simulink model "dynamicANN"  (R2019b)
settings: Solver=VariableStepAuto  StartTime=0.0  StopTime=3  RelTol=1e-3
values from neighbouring files (symbols this model uses):
  a = 87.548e-3    (= 0.087548)    [main.m]
  b = 132.452e-3    (= 0.132452)    [main.m]
  d = 22.452e-3    (= 0.022452)    [main.m]
  delta = 4e-6    (= 4e-06)    [main.m]
  F1 = mass*g-F2    (= 23.4474357109)    [main.m]
  F2 = a*mass*g/(a+b)    (= 15.4982642891)    [main.m]
  g = 9.81    [main.m]
  h0 = 75e-6    (= 7.5e-05)    [main.m]
  Jd = 0.047331604    [main.m]
  Jp = 0.00075    [main.m]
  Kps = (Vmax-Vmin)/(Hmax-Hmin)    (= 1666.66666667)    [main.m]
  Ksv = 30    [main.m]
  mass = 3.970    (= 3.97)    [main.m]
  mm = F2/g    (= 1.57984345455)    [main.m]
  omega = n_rpm*2*pi/60    (= 293.215314335)    [main.m]
  s = 30e-3    (= 0.03)    [main.m]
  tau = 0.12    [main.m]
  taus = 0.00125    [main.m]
  Ts = 1/fs    (= 0.001)    [main.m]
libraries: neural x480, simulink x2
(part 11 of 11)

== system dynamicANN/SERVOVALVES/HYDROSTATIC FORCES APPROXIMATION/Layer 2/LW{2,1} ==
  "ad{2,1}" : Inport  PortDimensions=50
      mask Display: e = 0.06;c1 = [120 230 180]/255;c2 = ([120 230 180]+0)/(256+128);c3 = ([120 230 180]+128)/(256+128);patch([0 1 1 0],[0 0 1 1],c1);patch([0 1 1 1-e 1-e 0+e],[0 0 1 1-e 0+e 0+e],c2);patch([0 0 1 1-e 0+e 0+e],[0 1 1 1-e 1-e 0+e],c3);plot([0 1 1 0 0],[0 0 1 1 0]);
  "IW{2,1}(1,:)'" : Constant  Value=[-1.014165171456560710083749654586426913738250732421875;0.74254120405114820702152655940153636038303375244140625;-0.493657103560888099735848300042562186717987060546875;1.762347654234217575464072069735266268253326416015625;0.77261513991503283360628984155482612550258636474609375;0.318276655083587822758772745146416127681732177734375;0.4305854427140574092192082389374263584613800048828125;0.1184731097225189266897160678126965649425983428955078125;-0.438124466002386803165080664257402531802654266357421875;1.09137751006303229672766974545083940029144287109375;-0.490669166841488202379650829243473708629608154296875;-0.98834811164750779877152808694518171250820159912109375;1.0590431490617298049272676507825963199138641357421875;-1.776082676108671432047003690968267619609832763671875;-2.06612743120169906063665621331892907619476318359375;-0.64589634160559905584619855289929546415805816650390625;-0.4327766588303278982863275814452208578586578369140625;-1.727153899806108672265736458939500153064727783203125;0.59181904704496124391965850009000860154628753662109375;0.16959741359399671534191611499409191310405731201171875;0.67424149151247203537451468946528621017932891845703125;0.585530221611660461888959616771899163722991943359375;1.0280769199996886431591747168567962944507598876953125;-0.2953895750385611140842456734389998018741607666015625;-0.288245131766746875978668640527757816016674041748046875;1.3110256721162059090346474476973526179790496826171875;-0.94479089477446398515070313806063495576381683349609375;2.976859202869103881994305993430316448211669921875;1.00813878716374727417814938235096633434295654296875;0.55045191126284465088502884100307710468769073486328125;-0.402896139933797303722684546301024965941905975341796875;0.6531782510692634158289138213149271905422210693359375;-0.339620575450382045090691462974064052104949951171875;-1.548768075257708431990977260284125804901123046875;-0.1751011740113746217861745435584452934563159942626953125;-1.493850957399413648118979835999198257923126220703125;-0.414405881298872402762611955040483735501766204833984375;1.3784631005445773244133533808053471148014068603515625;0.43496611827169628927691746866912581026554107666015625;1.2371551637692241865096320907468907535076141357421875;-0.429415029853276120075378230467322282493114471435546875;0.72610511484034712115231968709849752485752105712890625;0.528784547083847922266386376577429473400115966796875;-0.355625475679885505453370342365815304219722747802734375;-0.81546763135191124849399102458846755325794219970703125;-0.43196629902076733031890398706309497356414794921875;2.141633472647410219025232436251826584339141845703125;-0.942809116362634203056813930743373930454254150390625;0.50673484573840033018399253705865703523159027099609375;-0.311824293494437132512331345424172468483448028564453125]
      mask Display: e = 0.06;c1 = [120 150 230]/255;c2 = ([120 150 230]+0)/383;c3 = ([120 150 230]+128)/383;patch([0 1 1 0],[0 0 1 1],c1);patch([0 1 1 1-e 1-e 0+e],[0 0 1 1-e 0+e 0+e],c2);patch([0 0 1 1-e 0+e 0+e],[0 1 1 1-e 1-e 0+e],c3);plot([0 1 1 0 0],[0 0 1 1 0]);disp('weights');
  "IW{2,1}(2,:)'" : Constant  Value=[3.02639673612086568255108431912958621978759765625;0.7885923810484214424576521196286194026470184326171875;-2.164530907189261110801226095645688474178314208984375;-0.245729748797801850201949491747654974460601806640625;-0.00808531557296920423694164270500550628639757633209228515625;-0.76387022351862265967525900123291648924350738525390625;0.0827290827070368550710810495729674585163593292236328125;-0.6097012388277927019686330822878517210483551025390625;-0.74928046916180968128884387624566443264484405517578125;2.951882377774577737028494084370322525501251220703125;-2.1842359326909264183314007823355495929718017578125;2.530648543456691879072195661137811839580535888671875;3.18021236840055276928751482046209275722503662109375;0.14051115708063510734149303971207700669765472412109375;0.06445474728021070853767326980232610367238521575927734375;1.457545283477658326631853924482129514217376708984375;-1.621429868292408205121546416194178164005279541015625;0.279376315092421834140878900143434293568134307861328125;-0.8789785739954181220667805973789654672145843505859375;1.3220455668841974983251930098049342632293701171875;1.933304350227246004578773863613605499267578125;1.098485890073359172447453602217137813568115234375;-1.50724817303466007700762929744087159633636474609375;-0.6862057691770095946282026488916017115116119384765625;-1.1824579770952807766803971389890648424625396728515625;-1.294521403451049490485047499532811343669891357421875;0.435494894476214755574261516812839545309543609619140625;-1.1980880870527113035706179289263673126697540283203125;-0.29411642131463688887293983498238958418369293212890625;-0.5801295069320904218557188869453966617584228515625;0.00783844178986191353342150023308931849896907806396484375;0.64151166497871681126952125850948505103588104248046875;-0.580909108960366182827783632092177867889404296875;-1.5317767480030484161801496156840585172176361083984375;-1.55665554144854834106581620289944112300872802734375;-1.444847369615960275268662371672689914703369140625;-1.3425084490430860828524828320951201021671295166015625;-0.5131835470496282081143135656020604074001312255859375;0.764211347515264538543533490155823528766632080078125;-0.1667272900532859314370881520517286844551563262939453125;1.6458130141065983043091591753182001411914825439453125;-0.2219392160808244252034882038060459308326244354248046875;1.6264036561568058214533039063098840415477752685546875;-0.18886871647990266520622526513761840760707855224609375;-0.728706117737796699174168679746799170970916748046875;-2.016403595037946860912825286504812538623809814453125;0.029398033365513019654624571330714388750493526458740234375;-2.93245822543744250054942312999628484249114990234375;3.147405101749385369913625254412181675434112548828125;1.4208462681749429723510047551826573908329010009765625]
      mask Display: e = 0.06;c1 = [120 150 230]/255;c2 = ([120 150 230]+0)/383;c3 = ([120 150 230]+128)/383;patch([0 1 1 0],[0 0 1 1],c1);patch([0 1 1 1-e 1-e 0+e],[0 0 1 1-e 0+e 0+e],c2);patch([0 0 1 1-e 0+e 0+e],[0 1 1 1-e 1-e 0+e],c3);plot([0 1 1 0 0],[0 0 1 1 0]);disp('weights');
  Mux : Mux  Inputs=2
      mask Display: e = 0.06;c1 = [120 150 230]/255;c2 = ([120 150 230]+0)/383;c3 = ([120 150 230]+128)/383;patch([0 1 1 0],[0 0 1 1],c1);patch([0 1 1 1-e 1-e 0+e],[0 0 1 1-e 0+e 0+e],c2);patch([0 0 1 1-e 0+e 0+e],[0 1 1 1-e 1-e 0+e],c3);plot([0 1 1 0 0],[0 0 1 1 0]);disp('Mux');
  dotprod1 : neural/Weight Functions/dotprod
      settings: SourceProductName=Deep Learning Toolbox
  dotprod2 : neural/Weight Functions/dotprod
      settings: SourceProductName=Deep Learning Toolbox
  "lz{2,1}" : Outport
      mask Display: e = 0.06;c1 = [120 230 180]/255;c2 = ([120 230 180]+0)/(256+128);c3 = ([120 230 180]+128)/(256+128);patch([0 1 1 0],[0 0 1 1],c1);patch([0 1 1 1-e 1-e 0+e],[0 0 1 1-e 0+e 0+e],c2);patch([0 0 1 1-e 0+e 0+e],[0 1 1 1-e 1-e 0+e],c3);plot([0 1 1 0 0],[0 0 1 1 0]);
  wires:
  "IW{2,1}(1,:)'"/1 -> dotprod1/1
  "ad{2,1}"/1 -> dotprod1/2, dotprod2/2
  dotprod1/1 -> Mux/1
  "IW{2,1}(2,:)'"/1 -> dotprod2/1
  dotprod2/1 -> Mux/2
  Mux/1 -> "lz{2,1}"/1

== matlab function dynamicANN/REFERENCE SHAPING (cos) ==
  data: t input; t0 input; t1 input; Xc input; REFX output; Yc input; Xref input; Yref input; REFY output
function [REFX, REFY] = RefShaping(t,t0,t1,Xc,Yc,Xref,Yref)
Ax=(Xref-Xc)/2;
Ay=(Yref-Yc)/2;
w=pi/(t1-t0);

if t<t0
    REFX=Xc;
    REFY=Yc;
else if t>t1
        REFX=Xref;
        REFY=Yref;
    else
        REFX=Ax*cos(w*(t-t0)+pi)+(Xc+Ax);
        REFY=Ay*cos(w*(t-t0)+pi)+(Yc+Ay);
    end
end

== matlab function dynamicANN/STEP REFERENCE ==
  data: t input; t0 input; Xc input; REFX output; Yc input; Xref input; Yref input; REFY output
function [REFX, REFY] = StepReference(t,t0,Xc,Yc,Xref,Yref)
if t<t0
    REFX=Xc;
    REFY=Yc;
else
    REFX=Xref;
    REFY=Yref;
end
